simulink model "CoordinateTransform"  (R2025a)
settings: Solver=VariableStepAuto  StartTime=0.0  StopTime=1.0  RelTol=1e-3
undefined symbols (not defined in the file): DiscIntNeverNeededParam
libraries: simulink x2
settings Model: Creator=jicai  LastModifiedBy=jicai

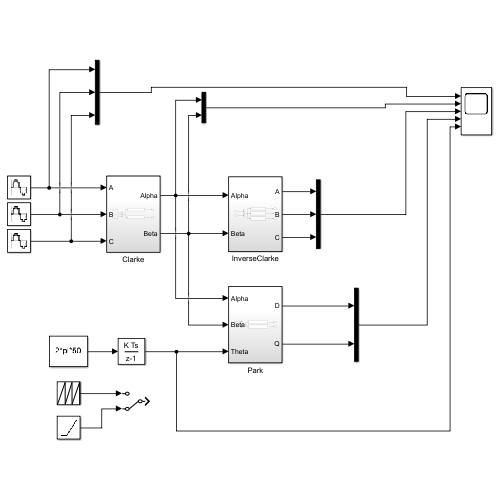
[thumbnail: Simulink's stored preview of the top-level diagram]
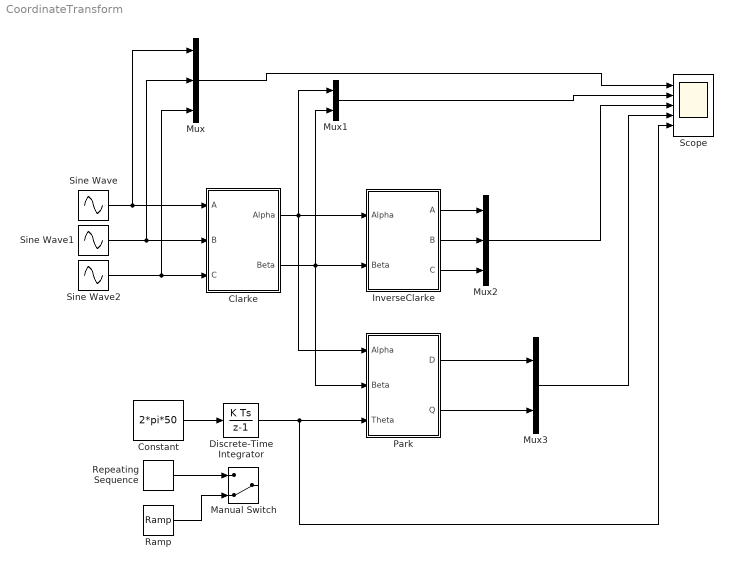
== system CoordinateTransform ==
  Clarke : Subsystem
  Constant : Constant  Value=2*pi*50  SampleTime=0.00001
  Discrete-Time Integrator : DiscreteIntegrator  SampleTime=0.00001  LowerSaturationLimit=inf  ICPrevOutput=DiscIntNeverNeededParam  ICPrevScaledInput=DiscIntNeverNeededParam
  InverseClarke : Subsystem
  Manual Switch : ManualSwitch  CurrentSetting=0
  Mux : Mux  Inputs=3
  Mux1 : Mux  Inputs=2
  Mux2 : Mux  Inputs=3
  Mux3 : Mux  Inputs=2
  Park : Subsystem
  Ramp : simulink/Sources/Ramp  slope=100*pi  start=0  InitialOutput=0
  Repeating Sequence : simulink/Sources/Repeating Sequence  rep_seq_t=[0 1]  rep_seq_y=[0 2*pi*50]
  Scope : Scope  NumInputPorts=5
      settings: ActiveDisplayString=5  Title=Theta  ActiveDisplayYMinimum=-39.258912595563942  ActiveDisplayYMaximum=353.33021336007556
  Sine Wave : Sin  Amplitude=100  Frequency=2*pi*50  SampleTime=0.00001
  Sine Wave1 : Sin  Amplitude=100  Frequency=2*pi*50  Phase=-pi*2/3  SampleTime=0.00001
  Sine Wave2 : Sin  Amplitude=100  Frequency=2*pi*50  Phase=pi*2/3  SampleTime=0.00001
  wires:
  Sine Wave/1 -> Mux/1, Clarke/1(A)
  Sine Wave1/1 -> Mux/2, Clarke/2(B)
  Sine Wave2/1 -> Mux/3, Clarke/3(C)
  Clarke/1(Alpha) -> Park/1(Alpha), Mux1/1, InverseClarke/1(Alpha)
  Clarke/2(Beta) -> Park/2(Beta), Mux1/2, InverseClarke/2(Beta)
  Mux/1 -> Scope/1
  Mux1/1 -> Scope/2
  InverseClarke/1(A) -> Mux2/1
  InverseClarke/2(B) -> Mux2/2
  InverseClarke/3(C) -> Mux2/3
  Mux2/1 -> Scope/3
  Constant/1 -> Discrete-Time Integrator/1
  Park/1(D) -> Mux3/1
  Park/2(Q) -> Mux3/2
  Mux3/1 -> Scope/4
  Repeating Sequence/1 -> Manual Switch/1
  Ramp/1 -> Manual Switch/2
  Discrete-Time Integrator/1 -> Park/3(Theta), Scope/5

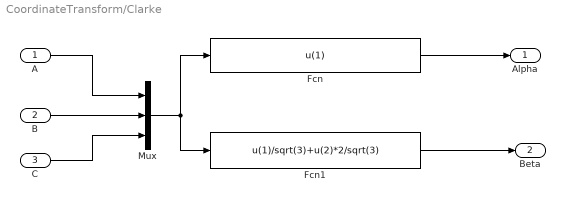
== system CoordinateTransform/Clarke ==
  A : Inport
  B : Inport  Port=2
  C : Inport  Port=3
  Fcn : Fcn  Expr=u(1)
  Fcn1 : Fcn  Expr=u(1)/sqrt(3)+u(2)*2/sqrt(3)
  Mux : Mux  Inputs=3
  Alpha : Outport
  Beta : Outport  Port=2
  wires:
  Mux/1 -> Fcn1/1, Fcn/1
  Fcn1/1 -> Beta/1
  Fcn/1 -> Alpha/1
  C/1 -> Mux/3
  A/1 -> Mux/1
  B/1 -> Mux/2

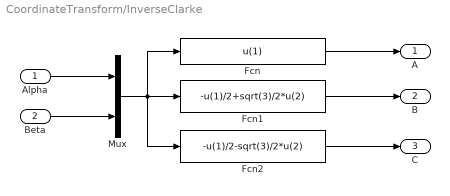
== system CoordinateTransform/InverseClarke ==
  Alpha : Inport
  Beta : Inport  Port=2
  Fcn : Fcn  Expr=u(1)
  Fcn1 : Fcn  Expr=-u(1)/2+sqrt(3)/2*u(2)
  Fcn2 : Fcn  Expr=-u(1)/2-sqrt(3)/2*u(2)
  Mux : Mux  Inputs=2
  A : Outport
  B : Outport  Port=2
  C : Outport  Port=3
  wires:
  Fcn2/1 -> C/1
  Alpha/1 -> Mux/1
  Mux/1 -> Fcn2/1, Fcn/1, Fcn1/1
  Fcn/1 -> A/1
  Beta/1 -> Mux/2
  Fcn1/1 -> B/1

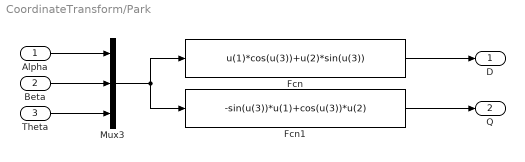
== system CoordinateTransform/Park ==
  Alpha : Inport
  Beta : Inport  Port=2
  Theta : Inport  Port=3
  Fcn : Fcn  Expr=u(1)*cos(u(3))+u(2)*sin(u(3))
  Fcn1 : Fcn  Expr=-sin(u(3))*u(1)+cos(u(3))*u(2)
  Mux3 : Mux  Inputs=3
  D : Outport
  Q : Outport  Port=2
  wires:
  Beta/1 -> Mux3/2
  Fcn/1 -> D/1
  Alpha/1 -> Mux3/1
  Theta/1 -> Mux3/3
  Fcn1/1 -> Q/1
  Mux3/1 -> Fcn1/1, Fcn/1
